simulink model "systemOffLine"  (Simulink 8.5)
settings: Solver=ode3  SolverMode=SingleTasking  StartTime=0.0  StopTime=0.1  RelTol=1e-3  AbsTol=1e-6
undefined symbols (not defined in the file or in its folder): DAB, den, elements, num
(part 5 of 5)

== system systemOffLine/Distance Relay Substation A2/Fault B-G Measurement/Zone R ==
  Z : Inport
  <V : Inport  Port=2
  " 5" : Fcn  Expr=sqrt(u)
  " 6" : RelationalOperator  Operator=<  OutDataTypeStr=boolean
  6 : Fcn  Expr=sqrt(u)
  Integrator : Integrator
  Product{,1..3} (4 alike) : Product  RndMeth=Zero
  "R, X" : Demux  Outputs=2
  Rdiff : Sum  Inputs=+-  SaturateOnIntegerOverflow=on  InputSameDT=on  OutDataTypeStr=Inherit: Same as first input
  Rr : Constant  Value=Rr/2
  Startup : Product  Inputs=3  RndMeth=Zero
  Step : Step  Time=0.017  SampleTime=0
  TRIP output contact : Relay  OnSwitchValue=0.9999  OffSwitchValue=-1
  Xdiff : Sum  Inputs=+-  SaturateOnIntegerOverflow=on  InputSameDT=on  OutDataTypeStr=Inherit: Same as first input
  Xr : Constant  Value=Xr/2
  Zm2 : Sum  SaturateOnIntegerOverflow=on  InputSameDT=on  OutDataTypeStr=Inherit: Same as first input
  Zr2 : Sum  SaturateOnIntegerOverflow=on  InputSameDT=on  OutDataTypeStr=Inherit: Same as first input
  delay : RelationalOperator  Operator=>  InputSameDT=on
  time delay : Constant  Value=Td+0.001
  TRIP : Outport  InitialOutput=0
  Zm : Outport  Port=2  InitialOutput=0
  Zr : Outport  Port=3  InitialOutput=0
  wires:
  Z/1 -> "R, X"/1
  Rr/1 -> Rdiff/1, Product1/2, Product1/1
  "R, X"/1 -> Rdiff/2
  "R, X"/2 -> Xdiff/1
  Xr/1 -> Xdiff/2, Product3/2, Product3/1
  Xdiff/1 -> Product2/2, Product2/1
  Product/1 -> Zm2/1
  Product2/1 -> Zm2/2
  Product1/1 -> Zr2/1
  Product3/1 -> Zr2/2
  Zm2/1 -> 6/1
  Zr2/1 -> " 5"/1
  6/1 -> " 6"/1, Zm/1
  " 5"/1 -> " 6"/2, Zr/1
  " 6"/1 -> Startup/1
  <V/1 -> Startup/3
  Step/1 -> Startup/2
  Rdiff/1 -> Product/1, Product/2
  Integrator/1 -> delay/1
  time delay/1 -> delay/2
  delay/1 -> TRIP output contact/1
  Startup/1 -> Integrator/1
  TRIP output contact/1 -> TRIP/1

== system systemOffLine/Distance Relay Substation A2/Fault C-A Measurement/Zone 1 ==
  Z : Inport
  <V : Inport  Port=2
  " 5" : Fcn  Expr=sqrt(u)
  " 6" : RelationalOperator  Operator=<  OutDataTypeStr=boolean
  6 : Fcn  Expr=sqrt(u)
  Integrator : Integrator
  Product{,1..3} (4 alike) : Product  RndMeth=Zero
  "R, X" : Demux  Outputs=2
  Rdiff : Sum  Inputs=+-  SaturateOnIntegerOverflow=on  InputSameDT=on  OutDataTypeStr=Inherit: Same as first input
  Rr : Constant  Value=Rr/2
  Startup : Product  Inputs=3  RndMeth=Zero
  Step : Step  Time=0.017  SampleTime=0
  TRIP output contact : Relay  OnSwitchValue=0.9999  OffSwitchValue=-1
  Xdiff : Sum  Inputs=+-  SaturateOnIntegerOverflow=on  InputSameDT=on  OutDataTypeStr=Inherit: Same as first input
  Xr : Constant  Value=Xr/2
  Zm2 : Sum  SaturateOnIntegerOverflow=on  InputSameDT=on  OutDataTypeStr=Inherit: Same as first input
  Zr2 : Sum  SaturateOnIntegerOverflow=on  InputSameDT=on  OutDataTypeStr=Inherit: Same as first input
  delay : RelationalOperator  Operator=>  InputSameDT=on
  time delay : Constant  Value=Td+0.001
  TRIP : Outport  InitialOutput=0
  Zm : Outport  Port=2  InitialOutput=0
  Zr : Outport  Port=3  InitialOutput=0
  wires:
  TRIP output contact/1 -> TRIP/1
  Startup/1 -> Integrator/1
  delay/1 -> TRIP output contact/1
  time delay/1 -> delay/2
  Integrator/1 -> delay/1
  Rdiff/1 -> Product/2, Product/1
  Step/1 -> Startup/2
  <V/1 -> Startup/3
  " 6"/1 -> Startup/1
  " 5"/1 -> Zr/1, " 6"/2
  6/1 -> Zm/1, " 6"/1
  Zr2/1 -> " 5"/1
  Zm2/1 -> 6/1
  Product3/1 -> Zr2/2
  Product1/1 -> Zr2/1
  Product2/1 -> Zm2/2
  Product/1 -> Zm2/1
  Xdiff/1 -> Product2/1, Product2/2
  Xr/1 -> Product3/1, Product3/2, Xdiff/2
  "R, X"/2 -> Xdiff/1
  "R, X"/1 -> Rdiff/2
  Rr/1 -> Product1/1, Product1/2, Rdiff/1
  Z/1 -> "R, X"/1

== system systemOffLine/Distance Relay Substation A2/Fault C-A Measurement/Zone 2 ==
  Z : Inport
  <V : Inport  Port=2
  " 5" : Fcn  Expr=sqrt(u)
  " 6" : RelationalOperator  Operator=<  OutDataTypeStr=boolean
  6 : Fcn  Expr=sqrt(u)
  Integrator : Integrator
  Product{,1..3} (4 alike) : Product  RndMeth=Zero
  "R, X" : Demux  Outputs=2
  Rdiff : Sum  Inputs=+-  SaturateOnIntegerOverflow=on  InputSameDT=on  OutDataTypeStr=Inherit: Same as first input
  Rr : Constant  Value=Rr/2
  Startup : Product  Inputs=3  RndMeth=Zero
  Step : Step  Time=0.017  SampleTime=0
  TRIP output contact : Relay  OnSwitchValue=0.9999  OffSwitchValue=-1
  Xdiff : Sum  Inputs=+-  SaturateOnIntegerOverflow=on  InputSameDT=on  OutDataTypeStr=Inherit: Same as first input
  Xr : Constant  Value=Xr/2
  Zm2 : Sum  SaturateOnIntegerOverflow=on  InputSameDT=on  OutDataTypeStr=Inherit: Same as first input
  Zr2 : Sum  SaturateOnIntegerOverflow=on  InputSameDT=on  OutDataTypeStr=Inherit: Same as first input
  delay : RelationalOperator  Operator=>  InputSameDT=on
  time delay : Constant  Value=Td+0.001
  TRIP : Outport  InitialOutput=0
  Zm : Outport  Port=2  InitialOutput=0
  Zr : Outport  Port=3  InitialOutput=0
  wires:
  Z/1 -> "R, X"/1
  Rr/1 -> Rdiff/1, Product1/2, Product1/1
  "R, X"/1 -> Rdiff/2
  "R, X"/2 -> Xdiff/1
  Xr/1 -> Xdiff/2, Product3/2, Product3/1
  Xdiff/1 -> Product2/2, Product2/1
  Product/1 -> Zm2/1
  Product2/1 -> Zm2/2
  Product1/1 -> Zr2/1
  Product3/1 -> Zr2/2
  Zm2/1 -> 6/1
  Zr2/1 -> " 5"/1
  6/1 -> " 6"/1, Zm/1
  " 5"/1 -> " 6"/2, Zr/1
  " 6"/1 -> Startup/1
  <V/1 -> Startup/3
  Step/1 -> Startup/2
  Rdiff/1 -> Product/1, Product/2
  Integrator/1 -> delay/1
  time delay/1 -> delay/2
  delay/1 -> TRIP output contact/1
  Startup/1 -> Integrator/1
  TRIP output contact/1 -> TRIP/1

== system systemOffLine/Distance Relay Substation A2/Fault C-A Measurement/Zone 3 ==
  Z : Inport
  <V : Inport  Port=2
  " 5" : Fcn  Expr=sqrt(u)
  " 6" : RelationalOperator  Operator=<  OutDataTypeStr=boolean
  6 : Fcn  Expr=sqrt(u)
  Integrator : Integrator
  Product{,1..3} (4 alike) : Product  RndMeth=Zero
  "R, X" : Demux  Outputs=2
  Rdiff : Sum  Inputs=+-  SaturateOnIntegerOverflow=on  InputSameDT=on  OutDataTypeStr=Inherit: Same as first input
  Rr : Constant  Value=-Rr/2
  Startup : Product  Inputs=3  RndMeth=Zero
  Step : Step  Time=0.017  SampleTime=0
  TRIP output contact : Relay  OnSwitchValue=0.9999  OffSwitchValue=-1
  Xdiff : Sum  Inputs=+-  SaturateOnIntegerOverflow=on  InputSameDT=on  OutDataTypeStr=Inherit: Same as first input
  Xr : Constant  Value=-Xr/2
  Zm2 : Sum  SaturateOnIntegerOverflow=on  InputSameDT=on  OutDataTypeStr=Inherit: Same as first input
  Zr2 : Sum  SaturateOnIntegerOverflow=on  InputSameDT=on  OutDataTypeStr=Inherit: Same as first input
  delay : RelationalOperator  Operator=>  InputSameDT=on
  time delay : Constant  Value=Td+0.001
  TRIP : Outport  InitialOutput=0
  Zm : Outport  Port=2  InitialOutput=0
  Zr : Outport  Port=3  InitialOutput=0
  wires:
  TRIP output contact/1 -> TRIP/1
  Startup/1 -> Integrator/1
  delay/1 -> TRIP output contact/1
  time delay/1 -> delay/2
  Integrator/1 -> delay/1
  Rdiff/1 -> Product/2, Product/1
  Step/1 -> Startup/2
  <V/1 -> Startup/3
  " 6"/1 -> Startup/1
  " 5"/1 -> Zr/1, " 6"/2
  6/1 -> Zm/1, " 6"/1
  Zr2/1 -> " 5"/1
  Zm2/1 -> 6/1
  Product3/1 -> Zr2/2
  Product1/1 -> Zr2/1
  Product2/1 -> Zm2/2
  Product/1 -> Zm2/1
  Xdiff/1 -> Product2/1, Product2/2
  Xr/1 -> Product3/1, Product3/2, Xdiff/2
  "R, X"/2 -> Xdiff/1
  "R, X"/1 -> Rdiff/2
  Rr/1 -> Product1/1, Product1/2, Rdiff/1
  Z/1 -> "R, X"/1

== system systemOffLine/Distance Relay Substation A2/Fault C-A Measurement/Zone 4 ==
  Z : Inport
  <V : Inport  Port=2
  " 5" : Fcn  Expr=sqrt(u)
  " 6" : RelationalOperator  Operator=<  OutDataTypeStr=boolean
  6 : Fcn  Expr=sqrt(u)
  Integrator : Integrator
  Product{,1..3} (4 alike) : Product  RndMeth=Zero
  "R, X" : Demux  Outputs=2
  Rdiff : Sum  Inputs=+-  SaturateOnIntegerOverflow=on  InputSameDT=on  OutDataTypeStr=Inherit: Same as first input
  Rr : Constant  Value=Rr/2
  Startup : Product  Inputs=3  RndMeth=Zero
  Step : Step  Time=0.017  SampleTime=0
  TRIP output contact : Relay  OnSwitchValue=0.9999  OffSwitchValue=-1
  Xdiff : Sum  Inputs=+-  SaturateOnIntegerOverflow=on  InputSameDT=on  OutDataTypeStr=Inherit: Same as first input
  Xr : Constant  Value=Xr/2
  Zm2 : Sum  SaturateOnIntegerOverflow=on  InputSameDT=on  OutDataTypeStr=Inherit: Same as first input
  Zr2 : Sum  SaturateOnIntegerOverflow=on  InputSameDT=on  OutDataTypeStr=Inherit: Same as first input
  delay : RelationalOperator  Operator=>  InputSameDT=on
  time delay : Constant  Value=Td+0.001
  TRIP : Outport  InitialOutput=0
  Zm : Outport  Port=2  InitialOutput=0
  Zr : Outport  Port=3  InitialOutput=0
  wires:
  Z/1 -> "R, X"/1
  Rr/1 -> Rdiff/1, Product1/2, Product1/1
  "R, X"/1 -> Rdiff/2
  "R, X"/2 -> Xdiff/1
  Xr/1 -> Xdiff/2, Product3/2, Product3/1
  Xdiff/1 -> Product2/2, Product2/1
  Product/1 -> Zm2/1
  Product2/1 -> Zm2/2
  Product1/1 -> Zr2/1
  Product3/1 -> Zr2/2
  Zm2/1 -> 6/1
  Zr2/1 -> " 5"/1
  6/1 -> " 6"/1, Zm/1
  " 5"/1 -> " 6"/2, Zr/1
  " 6"/1 -> Startup/1
  <V/1 -> Startup/3
  Step/1 -> Startup/2
  Rdiff/1 -> Product/1, Product/2
  Integrator/1 -> delay/1
  time delay/1 -> delay/2
  delay/1 -> TRIP output contact/1
  Startup/1 -> Integrator/1
  TRIP output contact/1 -> TRIP/1

== system systemOffLine/Distance Relay Substation A2/Fault C-A Measurement/Zone R ==
  Z : Inport
  <V : Inport  Port=2
  " 5" : Fcn  Expr=sqrt(u)
  " 6" : RelationalOperator  Operator=<  OutDataTypeStr=boolean
  6 : Fcn  Expr=sqrt(u)
  Integrator : Integrator
  Product{,1..3} (4 alike) : Product  RndMeth=Zero
  "R, X" : Demux  Outputs=2
  Rdiff : Sum  Inputs=+-  SaturateOnIntegerOverflow=on  InputSameDT=on  OutDataTypeStr=Inherit: Same as first input
  Rr : Constant  Value=Rr/2
  Startup : Product  Inputs=3  RndMeth=Zero
  Step : Step  Time=0.017  SampleTime=0
  TRIP output contact : Relay  OnSwitchValue=0.9999  OffSwitchValue=-1
  Xdiff : Sum  Inputs=+-  SaturateOnIntegerOverflow=on  InputSameDT=on  OutDataTypeStr=Inherit: Same as first input
  Xr : Constant  Value=Xr/2
  Zm2 : Sum  SaturateOnIntegerOverflow=on  InputSameDT=on  OutDataTypeStr=Inherit: Same as first input
  Zr2 : Sum  SaturateOnIntegerOverflow=on  InputSameDT=on  OutDataTypeStr=Inherit: Same as first input
  delay : RelationalOperator  Operator=>  InputSameDT=on
  time delay : Constant  Value=Td+0.001
  TRIP : Outport  InitialOutput=0
  Zm : Outport  Port=2  InitialOutput=0
  Zr : Outport  Port=3  InitialOutput=0
  wires:
  Z/1 -> "R, X"/1
  Rr/1 -> Rdiff/1, Product1/2, Product1/1
  "R, X"/1 -> Rdiff/2
  "R, X"/2 -> Xdiff/1
  Xr/1 -> Xdiff/2, Product3/2, Product3/1
  Xdiff/1 -> Product2/2, Product2/1
  Product/1 -> Zm2/1
  Product2/1 -> Zm2/2
  Product1/1 -> Zr2/1
  Product3/1 -> Zr2/2
  Zm2/1 -> 6/1
  Zr2/1 -> " 5"/1
  6/1 -> " 6"/1, Zm/1
  " 5"/1 -> " 6"/2, Zr/1
  " 6"/1 -> Startup/1
  <V/1 -> Startup/3
  Step/1 -> Startup/2
  Rdiff/1 -> Product/1, Product/2
  Integrator/1 -> delay/1
  time delay/1 -> delay/2
  delay/1 -> TRIP output contact/1
  Startup/1 -> Integrator/1
  TRIP output contact/1 -> TRIP/1

== system systemOffLine/Distance Relay Substation A2/Fault C-G Measurement/Zone 1 ==
  Z : Inport
  <V : Inport  Port=2
  " 5" : Fcn  Expr=sqrt(u)
  " 6" : RelationalOperator  Operator=<  OutDataTypeStr=boolean
  6 : Fcn  Expr=sqrt(u)
  Integrator : Integrator
  Product{,1..3} (4 alike) : Product  RndMeth=Zero
  "R, X" : Demux  Outputs=2
  Rdiff : Sum  Inputs=+-  SaturateOnIntegerOverflow=on  InputSameDT=on  OutDataTypeStr=Inherit: Same as first input
  Rr : Constant  Value=Rr/2
  Startup : Product  Inputs=3  RndMeth=Zero
  Step : Step  Time=0.017  SampleTime=0
  TRIP output contact : Relay  OnSwitchValue=0.9999  OffSwitchValue=-1
  Xdiff : Sum  Inputs=+-  SaturateOnIntegerOverflow=on  InputSameDT=on  OutDataTypeStr=Inherit: Same as first input
  Xr : Constant  Value=Xr/2
  Zm2 : Sum  SaturateOnIntegerOverflow=on  InputSameDT=on  OutDataTypeStr=Inherit: Same as first input
  Zr2 : Sum  SaturateOnIntegerOverflow=on  InputSameDT=on  OutDataTypeStr=Inherit: Same as first input
  delay : RelationalOperator  Operator=>  InputSameDT=on
  time delay : Constant  Value=Td+0.001
  TRIP : Outport  InitialOutput=0
  Zm : Outport  Port=2  InitialOutput=0
  Zr : Outport  Port=3  InitialOutput=0
  wires:
  TRIP output contact/1 -> TRIP/1
  Startup/1 -> Integrator/1
  delay/1 -> TRIP output contact/1
  time delay/1 -> delay/2
  Integrator/1 -> delay/1
  Rdiff/1 -> Product/2, Product/1
  Step/1 -> Startup/2
  <V/1 -> Startup/3
  " 6"/1 -> Startup/1
  " 5"/1 -> Zr/1, " 6"/2
  6/1 -> Zm/1, " 6"/1
  Zr2/1 -> " 5"/1
  Zm2/1 -> 6/1
  Product3/1 -> Zr2/2
  Product1/1 -> Zr2/1
  Product2/1 -> Zm2/2
  Product/1 -> Zm2/1
  Xdiff/1 -> Product2/1, Product2/2
  Xr/1 -> Product3/1, Product3/2, Xdiff/2
  "R, X"/2 -> Xdiff/1
  "R, X"/1 -> Rdiff/2
  Rr/1 -> Product1/1, Product1/2, Rdiff/1
  Z/1 -> "R, X"/1

== system systemOffLine/Distance Relay Substation A2/Fault C-G Measurement/Zone 2 ==
  Z : Inport
  <V : Inport  Port=2
  " 5" : Fcn  Expr=sqrt(u)
  " 6" : RelationalOperator  Operator=<  OutDataTypeStr=boolean
  6 : Fcn  Expr=sqrt(u)
  Integrator : Integrator
  Product{,1..3} (4 alike) : Product  RndMeth=Zero
  "R, X" : Demux  Outputs=2
  Rdiff : Sum  Inputs=+-  SaturateOnIntegerOverflow=on  InputSameDT=on  OutDataTypeStr=Inherit: Same as first input
  Rr : Constant  Value=Rr/2
  Startup : Product  Inputs=3  RndMeth=Zero
  Step : Step  Time=0.017  SampleTime=0
  TRIP output contact : Relay  OnSwitchValue=0.9999  OffSwitchValue=-1
  Xdiff : Sum  Inputs=+-  SaturateOnIntegerOverflow=on  InputSameDT=on  OutDataTypeStr=Inherit: Same as first input
  Xr : Constant  Value=Xr/2
  Zm2 : Sum  SaturateOnIntegerOverflow=on  InputSameDT=on  OutDataTypeStr=Inherit: Same as first input
  Zr2 : Sum  SaturateOnIntegerOverflow=on  InputSameDT=on  OutDataTypeStr=Inherit: Same as first input
  delay : RelationalOperator  Operator=>  InputSameDT=on
  time delay : Constant  Value=Td+0.001
  TRIP : Outport  InitialOutput=0
  Zm : Outport  Port=2  InitialOutput=0
  Zr : Outport  Port=3  InitialOutput=0
  wires:
  Z/1 -> "R, X"/1
  Rr/1 -> Rdiff/1, Product1/2, Product1/1
  "R, X"/1 -> Rdiff/2
  "R, X"/2 -> Xdiff/1
  Xr/1 -> Xdiff/2, Product3/2, Product3/1
  Xdiff/1 -> Product2/2, Product2/1
  Product/1 -> Zm2/1
  Product2/1 -> Zm2/2
  Product1/1 -> Zr2/1
  Product3/1 -> Zr2/2
  Zm2/1 -> 6/1
  Zr2/1 -> " 5"/1
  6/1 -> " 6"/1, Zm/1
  " 5"/1 -> " 6"/2, Zr/1
  " 6"/1 -> Startup/1
  <V/1 -> Startup/3
  Step/1 -> Startup/2
  Rdiff/1 -> Product/1, Product/2
  Integrator/1 -> delay/1
  time delay/1 -> delay/2
  delay/1 -> TRIP output contact/1
  Startup/1 -> Integrator/1
  TRIP output contact/1 -> TRIP/1

== system systemOffLine/Distance Relay Substation A2/Fault C-G Measurement/Zone 3 ==
  Z : Inport
  <V : Inport  Port=2
  " 5" : Fcn  Expr=sqrt(u)
  " 6" : RelationalOperator  Operator=<  OutDataTypeStr=boolean
  6 : Fcn  Expr=sqrt(u)
  Integrator : Integrator
  Product{,1..3} (4 alike) : Product  RndMeth=Zero
  "R, X" : Demux  Outputs=2
  Rdiff : Sum  Inputs=+-  SaturateOnIntegerOverflow=on  InputSameDT=on  OutDataTypeStr=Inherit: Same as first input
  Rr : Constant  Value=-Rr/2
  Startup : Product  Inputs=3  RndMeth=Zero
  Step : Step  Time=0.017  SampleTime=0
  TRIP output contact : Relay  OnSwitchValue=0.9999  OffSwitchValue=-1
  Xdiff : Sum  Inputs=+-  SaturateOnIntegerOverflow=on  InputSameDT=on  OutDataTypeStr=Inherit: Same as first input
  Xr : Constant  Value=-Xr/2
  Zm2 : Sum  SaturateOnIntegerOverflow=on  InputSameDT=on  OutDataTypeStr=Inherit: Same as first input
  Zr2 : Sum  SaturateOnIntegerOverflow=on  InputSameDT=on  OutDataTypeStr=Inherit: Same as first input
  delay : RelationalOperator  Operator=>  InputSameDT=on
  time delay : Constant  Value=Td+0.001
  TRIP : Outport  InitialOutput=0
  Zm : Outport  Port=2  InitialOutput=0
  Zr : Outport  Port=3  InitialOutput=0
  wires:
  TRIP output contact/1 -> TRIP/1
  Startup/1 -> Integrator/1
  delay/1 -> TRIP output contact/1
  time delay/1 -> delay/2
  Integrator/1 -> delay/1
  Rdiff/1 -> Product/2, Product/1
  Step/1 -> Startup/2
  <V/1 -> Startup/3
  " 6"/1 -> Startup/1
  " 5"/1 -> Zr/1, " 6"/2
  6/1 -> Zm/1, " 6"/1
  Zr2/1 -> " 5"/1
  Zm2/1 -> 6/1
  Product3/1 -> Zr2/2
  Product1/1 -> Zr2/1
  Product2/1 -> Zm2/2
  Product/1 -> Zm2/1
  Xdiff/1 -> Product2/1, Product2/2
  Xr/1 -> Product3/1, Product3/2, Xdiff/2
  "R, X"/2 -> Xdiff/1
  "R, X"/1 -> Rdiff/2
  Rr/1 -> Product1/1, Product1/2, Rdiff/1
  Z/1 -> "R, X"/1

== system systemOffLine/Distance Relay Substation A2/Fault C-G Measurement/Zone 4 ==
  Z : Inport
  <V : Inport  Port=2
  " 5" : Fcn  Expr=sqrt(u)
  " 6" : RelationalOperator  Operator=<  OutDataTypeStr=boolean
  6 : Fcn  Expr=sqrt(u)
  Integrator : Integrator
  Product{,1..3} (4 alike) : Product  RndMeth=Zero
  "R, X" : Demux  Outputs=2
  Rdiff : Sum  Inputs=+-  SaturateOnIntegerOverflow=on  InputSameDT=on  OutDataTypeStr=Inherit: Same as first input
  Rr : Constant  Value=Rr/2
  Startup : Product  Inputs=3  RndMeth=Zero
  Step : Step  Time=0.017  SampleTime=0
  TRIP output contact : Relay  OnSwitchValue=0.9999  OffSwitchValue=-1
  Xdiff : Sum  Inputs=+-  SaturateOnIntegerOverflow=on  InputSameDT=on  OutDataTypeStr=Inherit: Same as first input
  Xr : Constant  Value=Xr/2
  Zm2 : Sum  SaturateOnIntegerOverflow=on  InputSameDT=on  OutDataTypeStr=Inherit: Same as first input
  Zr2 : Sum  SaturateOnIntegerOverflow=on  InputSameDT=on  OutDataTypeStr=Inherit: Same as first input
  delay : RelationalOperator  Operator=>  InputSameDT=on
  time delay : Constant  Value=Td+0.001
  TRIP : Outport  InitialOutput=0
  Zm : Outport  Port=2  InitialOutput=0
  Zr : Outport  Port=3  InitialOutput=0
  wires:
  Z/1 -> "R, X"/1
  Rr/1 -> Rdiff/1, Product1/2, Product1/1
  "R, X"/1 -> Rdiff/2
  "R, X"/2 -> Xdiff/1
  Xr/1 -> Xdiff/2, Product3/2, Product3/1
  Xdiff/1 -> Product2/2, Product2/1
  Product/1 -> Zm2/1
  Product2/1 -> Zm2/2
  Product1/1 -> Zr2/1
  Product3/1 -> Zr2/2
  Zm2/1 -> 6/1
  Zr2/1 -> " 5"/1
  6/1 -> " 6"/1, Zm/1
  " 5"/1 -> " 6"/2, Zr/1
  " 6"/1 -> Startup/1
  <V/1 -> Startup/3
  Step/1 -> Startup/2
  Rdiff/1 -> Product/1, Product/2
  Integrator/1 -> delay/1
  time delay/1 -> delay/2
  delay/1 -> TRIP output contact/1
  Startup/1 -> Integrator/1
  TRIP output contact/1 -> TRIP/1

== system systemOffLine/Distance Relay Substation A2/Fault C-G Measurement/Zone R ==
  Z : Inport
  <V : Inport  Port=2
  " 5" : Fcn  Expr=sqrt(u)
  " 6" : RelationalOperator  Operator=<  OutDataTypeStr=boolean
  6 : Fcn  Expr=sqrt(u)
  Integrator : Integrator
  Product{,1..3} (4 alike) : Product  RndMeth=Zero
  "R, X" : Demux  Outputs=2
  Rdiff : Sum  Inputs=+-  SaturateOnIntegerOverflow=on  InputSameDT=on  OutDataTypeStr=Inherit: Same as first input
  Rr : Constant  Value=Rr/2
  Startup : Product  Inputs=3  RndMeth=Zero
  Step : Step  Time=0.017  SampleTime=0
  TRIP output contact : Relay  OnSwitchValue=0.9999  OffSwitchValue=-1
  Xdiff : Sum  Inputs=+-  SaturateOnIntegerOverflow=on  InputSameDT=on  OutDataTypeStr=Inherit: Same as first input
  Xr : Constant  Value=Xr/2
  Zm2 : Sum  SaturateOnIntegerOverflow=on  InputSameDT=on  OutDataTypeStr=Inherit: Same as first input
  Zr2 : Sum  SaturateOnIntegerOverflow=on  InputSameDT=on  OutDataTypeStr=Inherit: Same as first input
  delay : RelationalOperator  Operator=>  InputSameDT=on
  time delay : Constant  Value=Td+0.001
  TRIP : Outport  InitialOutput=0
  Zm : Outport  Port=2  InitialOutput=0
  Zr : Outport  Port=3  InitialOutput=0
  wires:
  Z/1 -> "R, X"/1
  Rr/1 -> Rdiff/1, Product1/2, Product1/1
  "R, X"/1 -> Rdiff/2
  "R, X"/2 -> Xdiff/1
  Xr/1 -> Xdiff/2, Product3/2, Product3/1
  Xdiff/1 -> Product2/2, Product2/1
  Product/1 -> Zm2/1
  Product2/1 -> Zm2/2
  Product1/1 -> Zr2/1
  Product3/1 -> Zr2/2
  Zm2/1 -> 6/1
  Zr2/1 -> " 5"/1
  6/1 -> " 6"/1, Zm/1
  " 5"/1 -> " 6"/2, Zr/1
  " 6"/1 -> Startup/1
  <V/1 -> Startup/3
  Step/1 -> Startup/2
  Rdiff/1 -> Product/1, Product/2
  Integrator/1 -> delay/1
  time delay/1 -> delay/2
  delay/1 -> TRIP output contact/1
  Startup/1 -> Integrator/1
  TRIP output contact/1 -> TRIP/1

== system systemOffLine/Distance Relay Substation A1/Analog filtering, signal  conditioning/CURRENTS/DAB - current A ==
  a : Inport
  Analog Filter : TransferFcn  Numerator=num  Denominator=den
  Gain : Gain  Gain=G  SaturateOnIntegerOverflow=on  OutDataTypeStr=Inherit: Same as input  ParamDataTypeStr=Inherit: Same as input
  d : Outport  InitialOutput=[zeros(winsize,1)]
  wires:
  a/1 -> Analog Filter/1
  Analog Filter/1 -> Gain/1
  Gain/1 -> d/1

== system systemOffLine/Distance Relay Substation A1/Analog filtering, signal  conditioning/CURRENTS/DAB - current B ==
  a : Inport
  Analog Filter : TransferFcn  Numerator=num  Denominator=den
  Gain : Gain  Gain=G  SaturateOnIntegerOverflow=on  OutDataTypeStr=Inherit: Same as input  ParamDataTypeStr=Inherit: Same as input
  d : Outport  InitialOutput=[zeros(winsize,1)]
  wires:
  Gain/1 -> d/1
  Analog Filter/1 -> Gain/1
  a/1 -> Analog Filter/1

== system systemOffLine/Distance Relay Substation A1/Analog filtering, signal  conditioning/CURRENTS/DAB - current C ==
  a : Inport
  Analog Filter : TransferFcn  Numerator=num  Denominator=den
  Gain : Gain  Gain=G  SaturateOnIntegerOverflow=on  OutDataTypeStr=Inherit: Same as input  ParamDataTypeStr=Inherit: Same as input
  d : Outport  InitialOutput=[zeros(winsize,1)]
  wires:
  a/1 -> Analog Filter/1
  Analog Filter/1 -> Gain/1
  Gain/1 -> d/1

== system systemOffLine/Distance Relay Substation A1/Analog filtering, signal  conditioning/CURRENTS/Phasor IA ==
  signal : Inport
  Fcn : Fcn  Expr=u^2
  Fcn1 : Fcn  Expr=u^2
  Fcn2 : Fcn  Expr=sqrt(u)
  Fcn3 : Fcn  Expr=180/pi*atan2(u[2],u[1])
  Gain1 : Gain  Gain=k*f1  SaturateOnIntegerOverflow=on  OutDataTypeStr=Inherit: Same as input  ParamDataTypeStr=Inherit: Same as input
  Integ2 : Integrator
  Mux : Mux  Inputs=2
  Product : Product  SaturateOnIntegerOverflow=on  InputSameDT=on  OutDataTypeStr=Inherit: Same as first input
  Product1 : Product  SaturateOnIntegerOverflow=on  InputSameDT=on  OutDataTypeStr=Inherit: Same as first input
  Sum : Sum  SaturateOnIntegerOverflow=on  InputSameDT=on  OutDataTypeStr=Inherit: Same as first input
  Sum1 : Sum  Inputs=+-  SaturateOnIntegerOverflow=on  InputSameDT=on  OutDataTypeStr=Inherit: Same as first input
  Sum2 : Sum  Inputs=+-  SaturateOnIntegerOverflow=on  InputSameDT=on  OutDataTypeStr=Inherit: Same as first input
  T1 : TransportDelay  DelayTime=1/f1  BufferSize=15360
  T2 : TransportDelay  DelayTime=1/f1  BufferSize=15360
  cos(nwt) : Sin  Frequency=2*pi*n*f1  Phase=pi/2  SampleTime=0
  integ1 : Integrator
  sin(nwt) : Sin  Frequency=2*pi*n*f1  SampleTime=0
  magnitude : Outport  InitialOutput=0
  angle : Outport  Port=2  InitialOutput=0
  wires:
  Sum/1 -> Fcn2/1
  Fcn/1 -> Sum/1
  Fcn1/1 -> Sum/2
  Mux/1 -> Fcn3/1
  Fcn3/1 -> angle/1
  sin(nwt)/1 -> Product/1
  cos(nwt)/1 -> Product1/2
  Product/1 -> integ1/1
  Product1/1 -> Integ2/1
  T1/1 -> Sum1/2
  T2/1 -> Sum2/2
  integ1/1 -> T1/1, Sum1/1
  Integ2/1 -> T2/1, Sum2/1
  Sum2/1 -> Fcn1/1, Mux/2
  Sum1/1 -> Fcn/1, Mux/1
  signal/1 -> Gain1/1
  Gain1/1 -> Product/2, Product1/1
  Fcn2/1 -> magnitude/1

== system systemOffLine/Distance Relay Substation A1/Analog filtering, signal  conditioning/CURRENTS/Phasor IB ==
  signal : Inport
  Fcn : Fcn  Expr=u^2
  Fcn1 : Fcn  Expr=u^2
  Fcn2 : Fcn  Expr=sqrt(u)
  Fcn3 : Fcn  Expr=180/pi*atan2(u[2],u[1])
  Gain1 : Gain  Gain=k*f1  SaturateOnIntegerOverflow=on  OutDataTypeStr=Inherit: Same as input  ParamDataTypeStr=Inherit: Same as input
  Integ2 : Integrator
  Mux : Mux  Inputs=2
  Product : Product  SaturateOnIntegerOverflow=on  InputSameDT=on  OutDataTypeStr=Inherit: Same as first input
  Product1 : Product  SaturateOnIntegerOverflow=on  InputSameDT=on  OutDataTypeStr=Inherit: Same as first input
  Sum : Sum  SaturateOnIntegerOverflow=on  InputSameDT=on  OutDataTypeStr=Inherit: Same as first input
  Sum1 : Sum  Inputs=+-  SaturateOnIntegerOverflow=on  InputSameDT=on  OutDataTypeStr=Inherit: Same as first input
  Sum2 : Sum  Inputs=+-  SaturateOnIntegerOverflow=on  InputSameDT=on  OutDataTypeStr=Inherit: Same as first input
  T1 : TransportDelay  DelayTime=1/f1  BufferSize=15360
  T2 : TransportDelay  DelayTime=1/f1  BufferSize=15360
  cos(nwt) : Sin  Frequency=2*pi*n*f1  Phase=pi/2  SampleTime=0
  integ1 : Integrator
  sin(nwt) : Sin  Frequency=2*pi*n*f1  SampleTime=0
  magnitude : Outport  InitialOutput=0
  angle : Outport  Port=2  InitialOutput=0
  wires:
  Fcn2/1 -> magnitude/1
  Gain1/1 -> Product1/1, Product/2
  signal/1 -> Gain1/1
  Sum1/1 -> Mux/1, Fcn/1
  Sum2/1 -> Mux/2, Fcn1/1
  Integ2/1 -> Sum2/1, T2/1
  integ1/1 -> Sum1/1, T1/1
  T2/1 -> Sum2/2
  T1/1 -> Sum1/2
  Product1/1 -> Integ2/1
  Product/1 -> integ1/1
  cos(nwt)/1 -> Product1/2
  sin(nwt)/1 -> Product/1
  Fcn3/1 -> angle/1
  Mux/1 -> Fcn3/1
  Fcn1/1 -> Sum/2
  Fcn/1 -> Sum/1
  Sum/1 -> Fcn2/1

== system systemOffLine/Distance Relay Substation A1/Analog filtering, signal  conditioning/CURRENTS/Phasor IC ==
  signal : Inport
  Fcn : Fcn  Expr=u^2
  Fcn1 : Fcn  Expr=u^2
  Fcn2 : Fcn  Expr=sqrt(u)
  Fcn3 : Fcn  Expr=180/pi*atan2(u[2],u[1])
  Gain1 : Gain  Gain=k*f1  SaturateOnIntegerOverflow=on  OutDataTypeStr=Inherit: Same as input  ParamDataTypeStr=Inherit: Same as input
  Integ2 : Integrator
  Mux : Mux  Inputs=2
  Product : Product  SaturateOnIntegerOverflow=on  InputSameDT=on  OutDataTypeStr=Inherit: Same as first input
  Product1 : Product  SaturateOnIntegerOverflow=on  InputSameDT=on  OutDataTypeStr=Inherit: Same as first input
  Sum : Sum  SaturateOnIntegerOverflow=on  InputSameDT=on  OutDataTypeStr=Inherit: Same as first input
  Sum1 : Sum  Inputs=+-  SaturateOnIntegerOverflow=on  InputSameDT=on  OutDataTypeStr=Inherit: Same as first input
  Sum2 : Sum  Inputs=+-  SaturateOnIntegerOverflow=on  InputSameDT=on  OutDataTypeStr=Inherit: Same as first input
  T1 : TransportDelay  DelayTime=1/f1  BufferSize=15360
  T2 : TransportDelay  DelayTime=1/f1  BufferSize=15360
  cos(nwt) : Sin  Frequency=2*pi*n*f1  Phase=pi/2  SampleTime=0
  integ1 : Integrator
  sin(nwt) : Sin  Frequency=2*pi*n*f1  SampleTime=0
  magnitude : Outport  InitialOutput=0
  angle : Outport  Port=2  InitialOutput=0
  wires:
  Sum/1 -> Fcn2/1
  Fcn/1 -> Sum/1
  Fcn1/1 -> Sum/2
  Mux/1 -> Fcn3/1
  Fcn3/1 -> angle/1
  sin(nwt)/1 -> Product/1
  cos(nwt)/1 -> Product1/2
  Product/1 -> integ1/1
  Product1/1 -> Integ2/1
  T1/1 -> Sum1/2
  T2/1 -> Sum2/2
  integ1/1 -> T1/1, Sum1/1
  Integ2/1 -> T2/1, Sum2/1
  Sum2/1 -> Fcn1/1, Mux/2
  Sum1/1 -> Fcn/1, Mux/1
  signal/1 -> Gain1/1
  Gain1/1 -> Product/2, Product1/1
  Fcn2/1 -> magnitude/1

== system systemOffLine/Distance Relay Substation A1/Analog filtering, signal  conditioning/VOLTAGES/DAB - voltage A ==
  a : Inport
  Analog Filter : TransferFcn  Numerator=num  Denominator=den
  Gain : Gain  Gain=G  SaturateOnIntegerOverflow=on  OutDataTypeStr=Inherit: Same as input  ParamDataTypeStr=Inherit: Same as input
  d : Outport  InitialOutput=[zeros(winsize,1)]
  wires:
  Gain/1 -> d/1
  Analog Filter/1 -> Gain/1
  a/1 -> Analog Filter/1

== system systemOffLine/Distance Relay Substation A1/Analog filtering, signal  conditioning/VOLTAGES/DAB - voltage B ==
  a : Inport
  Analog Filter : TransferFcn  Numerator=num  Denominator=den
  Gain : Gain  Gain=G  SaturateOnIntegerOverflow=on  OutDataTypeStr=Inherit: Same as input  ParamDataTypeStr=Inherit: Same as input
  d : Outport  InitialOutput=[zeros(winsize,1)]
  wires:
  a/1 -> Analog Filter/1
  Analog Filter/1 -> Gain/1
  Gain/1 -> d/1

== system systemOffLine/Distance Relay Substation A1/Analog filtering, signal  conditioning/VOLTAGES/DAB - voltage C ==
  a : Inport
  Analog Filter : TransferFcn  Numerator=num  Denominator=den
  Gain : Gain  Gain=G  SaturateOnIntegerOverflow=on  OutDataTypeStr=Inherit: Same as input  ParamDataTypeStr=Inherit: Same as input
  d : Outport  InitialOutput=[zeros(winsize,1)]
  wires:
  Gain/1 -> d/1
  Analog Filter/1 -> Gain/1
  a/1 -> Analog Filter/1

== system systemOffLine/Distance Relay Substation A1/Analog filtering, signal  conditioning/VOLTAGES/Phasor VA ==
  signal : Inport
  Fcn : Fcn  Expr=u^2
  Fcn1 : Fcn  Expr=u^2
  Fcn2 : Fcn  Expr=sqrt(u)
  Fcn3 : Fcn  Expr=180/pi*atan2(u[2],u[1])
  Gain1 : Gain  Gain=k*f1  SaturateOnIntegerOverflow=on  OutDataTypeStr=Inherit: Same as input  ParamDataTypeStr=Inherit: Same as input
  Integ2 : Integrator
  Mux : Mux  Inputs=2
  Product : Product  SaturateOnIntegerOverflow=on  InputSameDT=on  OutDataTypeStr=Inherit: Same as first input
  Product1 : Product  SaturateOnIntegerOverflow=on  InputSameDT=on  OutDataTypeStr=Inherit: Same as first input
  Sum : Sum  SaturateOnIntegerOverflow=on  InputSameDT=on  OutDataTypeStr=Inherit: Same as first input
  Sum1 : Sum  Inputs=+-  SaturateOnIntegerOverflow=on  InputSameDT=on  OutDataTypeStr=Inherit: Same as first input
  Sum2 : Sum  Inputs=+-  SaturateOnIntegerOverflow=on  InputSameDT=on  OutDataTypeStr=Inherit: Same as first input
  T1 : TransportDelay  DelayTime=1/f1  BufferSize=15360
  T2 : TransportDelay  DelayTime=1/f1  BufferSize=15360
  cos(nwt) : Sin  Frequency=2*pi*n*f1  Phase=pi/2  SampleTime=0
  integ1 : Integrator
  sin(nwt) : Sin  Frequency=2*pi*n*f1  SampleTime=0
  magnitude : Outport  InitialOutput=0
  angle : Outport  Port=2  InitialOutput=0
  wires:
  Sum/1 -> Fcn2/1
  Fcn/1 -> Sum/1
  Fcn1/1 -> Sum/2
  Mux/1 -> Fcn3/1
  Fcn3/1 -> angle/1
  sin(nwt)/1 -> Product/1
  cos(nwt)/1 -> Product1/2
  Product/1 -> integ1/1
  Product1/1 -> Integ2/1
  T1/1 -> Sum1/2
  T2/1 -> Sum2/2
  integ1/1 -> T1/1, Sum1/1
  Integ2/1 -> T2/1, Sum2/1
  Sum2/1 -> Fcn1/1, Mux/2
  Sum1/1 -> Fcn/1, Mux/1
  signal/1 -> Gain1/1
  Gain1/1 -> Product/2, Product1/1
  Fcn2/1 -> magnitude/1

== system systemOffLine/Distance Relay Substation A1/Analog filtering, signal  conditioning/VOLTAGES/Phasor VB ==
  signal : Inport
  Fcn : Fcn  Expr=u^2
  Fcn1 : Fcn  Expr=u^2
  Fcn2 : Fcn  Expr=sqrt(u)
  Fcn3 : Fcn  Expr=180/pi*atan2(u[2],u[1])
  Gain1 : Gain  Gain=k*f1  SaturateOnIntegerOverflow=on  OutDataTypeStr=Inherit: Same as input  ParamDataTypeStr=Inherit: Same as input
  Integ2 : Integrator
  Mux : Mux  Inputs=2
  Product : Product  SaturateOnIntegerOverflow=on  InputSameDT=on  OutDataTypeStr=Inherit: Same as first input
  Product1 : Product  SaturateOnIntegerOverflow=on  InputSameDT=on  OutDataTypeStr=Inherit: Same as first input
  Sum : Sum  SaturateOnIntegerOverflow=on  InputSameDT=on  OutDataTypeStr=Inherit: Same as first input
  Sum1 : Sum  Inputs=+-  SaturateOnIntegerOverflow=on  InputSameDT=on  OutDataTypeStr=Inherit: Same as first input
  Sum2 : Sum  Inputs=+-  SaturateOnIntegerOverflow=on  InputSameDT=on  OutDataTypeStr=Inherit: Same as first input
  T1 : TransportDelay  DelayTime=1/f1  BufferSize=15360
  T2 : TransportDelay  DelayTime=1/f1  BufferSize=15360
  cos(nwt) : Sin  Frequency=2*pi*n*f1  Phase=pi/2  SampleTime=0
  integ1 : Integrator
  sin(nwt) : Sin  Frequency=2*pi*n*f1  SampleTime=0
  magnitude : Outport  InitialOutput=0
  angle : Outport  Port=2  InitialOutput=0
  wires:
  Fcn2/1 -> magnitude/1
  Gain1/1 -> Product1/1, Product/2
  signal/1 -> Gain1/1
  Sum1/1 -> Mux/1, Fcn/1
  Sum2/1 -> Mux/2, Fcn1/1
  Integ2/1 -> Sum2/1, T2/1
  integ1/1 -> Sum1/1, T1/1
  T2/1 -> Sum2/2
  T1/1 -> Sum1/2
  Product1/1 -> Integ2/1
  Product/1 -> integ1/1
  cos(nwt)/1 -> Product1/2
  sin(nwt)/1 -> Product/1
  Fcn3/1 -> angle/1
  Mux/1 -> Fcn3/1
  Fcn1/1 -> Sum/2
  Fcn/1 -> Sum/1
  Sum/1 -> Fcn2/1

== system systemOffLine/Distance Relay Substation A1/Analog filtering, signal  conditioning/VOLTAGES/Phasor VC ==
  signal : Inport
  Fcn : Fcn  Expr=u^2
  Fcn1 : Fcn  Expr=u^2
  Fcn2 : Fcn  Expr=sqrt(u)
  Fcn3 : Fcn  Expr=180/pi*atan2(u[2],u[1])
  Gain1 : Gain  Gain=k*f1  SaturateOnIntegerOverflow=on  OutDataTypeStr=Inherit: Same as input  ParamDataTypeStr=Inherit: Same as input
  Integ2 : Integrator
  Mux : Mux  Inputs=2
  Product : Product  SaturateOnIntegerOverflow=on  InputSameDT=on  OutDataTypeStr=Inherit: Same as first input
  Product1 : Product  SaturateOnIntegerOverflow=on  InputSameDT=on  OutDataTypeStr=Inherit: Same as first input
  Sum : Sum  SaturateOnIntegerOverflow=on  InputSameDT=on  OutDataTypeStr=Inherit: Same as first input
  Sum1 : Sum  Inputs=+-  SaturateOnIntegerOverflow=on  InputSameDT=on  OutDataTypeStr=Inherit: Same as first input
  Sum2 : Sum  Inputs=+-  SaturateOnIntegerOverflow=on  InputSameDT=on  OutDataTypeStr=Inherit: Same as first input
  T1 : TransportDelay  DelayTime=1/f1  BufferSize=15360
  T2 : TransportDelay  DelayTime=1/f1  BufferSize=15360
  cos(nwt) : Sin  Frequency=2*pi*n*f1  Phase=pi/2  SampleTime=0
  integ1 : Integrator
  sin(nwt) : Sin  Frequency=2*pi*n*f1  SampleTime=0
  magnitude : Outport  InitialOutput=0
  angle : Outport  Port=2  InitialOutput=0
  wires:
  Sum/1 -> Fcn2/1
  Fcn/1 -> Sum/1
  Fcn1/1 -> Sum/2
  Mux/1 -> Fcn3/1
  Fcn3/1 -> angle/1
  sin(nwt)/1 -> Product/1
  cos(nwt)/1 -> Product1/2
  Product/1 -> integ1/1
  Product1/1 -> Integ2/1
  T1/1 -> Sum1/2
  T2/1 -> Sum2/2
  integ1/1 -> T1/1, Sum1/1
  Integ2/1 -> T2/1, Sum2/1
  Sum2/1 -> Fcn1/1, Mux/2
  Sum1/1 -> Fcn/1, Mux/1
  signal/1 -> Gain1/1
  Gain1/1 -> Product/2, Product1/1
  Fcn2/1 -> magnitude/1

== system systemOffLine/Distance Relay Substation A2/Analog filtering, signal  conditioning/CURRENTS/DAB - current A ==
  a : Inport
  Analog Filter : TransferFcn  Numerator=num  Denominator=den
  Gain : Gain  Gain=G  SaturateOnIntegerOverflow=on  OutDataTypeStr=Inherit: Same as input  ParamDataTypeStr=Inherit: Same as input
  d : Outport  InitialOutput=[zeros(winsize,1)]
  wires:
  a/1 -> Analog Filter/1
  Analog Filter/1 -> Gain/1
  Gain/1 -> d/1

== system systemOffLine/Distance Relay Substation A2/Analog filtering, signal  conditioning/CURRENTS/DAB - current B ==
  a : Inport
  Analog Filter : TransferFcn  Numerator=num  Denominator=den
  Gain : Gain  Gain=G  SaturateOnIntegerOverflow=on  OutDataTypeStr=Inherit: Same as input  ParamDataTypeStr=Inherit: Same as input
  d : Outport  InitialOutput=[zeros(winsize,1)]
  wires:
  Gain/1 -> d/1
  Analog Filter/1 -> Gain/1
  a/1 -> Analog Filter/1

== system systemOffLine/Distance Relay Substation A2/Analog filtering, signal  conditioning/CURRENTS/DAB - current C ==
  a : Inport
  Analog Filter : TransferFcn  Numerator=num  Denominator=den
  Gain : Gain  Gain=G  SaturateOnIntegerOverflow=on  OutDataTypeStr=Inherit: Same as input  ParamDataTypeStr=Inherit: Same as input
  d : Outport  InitialOutput=[zeros(winsize,1)]
  wires:
  a/1 -> Analog Filter/1
  Analog Filter/1 -> Gain/1
  Gain/1 -> d/1

== system systemOffLine/Distance Relay Substation A2/Analog filtering, signal  conditioning/CURRENTS/Phasor IA ==
  signal : Inport
  Fcn : Fcn  Expr=u^2
  Fcn1 : Fcn  Expr=u^2
  Fcn2 : Fcn  Expr=sqrt(u)
  Fcn3 : Fcn  Expr=180/pi*atan2(u[2],u[1])
  Gain1 : Gain  Gain=k*f1  SaturateOnIntegerOverflow=on  OutDataTypeStr=Inherit: Same as input  ParamDataTypeStr=Inherit: Same as input
  Integ2 : Integrator
  Mux : Mux  Inputs=2
  Product : Product  SaturateOnIntegerOverflow=on  InputSameDT=on  OutDataTypeStr=Inherit: Same as first input
  Product1 : Product  SaturateOnIntegerOverflow=on  InputSameDT=on  OutDataTypeStr=Inherit: Same as first input
  Sum : Sum  SaturateOnIntegerOverflow=on  InputSameDT=on  OutDataTypeStr=Inherit: Same as first input
  Sum1 : Sum  Inputs=+-  SaturateOnIntegerOverflow=on  InputSameDT=on  OutDataTypeStr=Inherit: Same as first input
  Sum2 : Sum  Inputs=+-  SaturateOnIntegerOverflow=on  InputSameDT=on  OutDataTypeStr=Inherit: Same as first input
  T1 : TransportDelay  DelayTime=1/f1  BufferSize=15360
  T2 : TransportDelay  DelayTime=1/f1  BufferSize=15360
  cos(nwt) : Sin  Frequency=2*pi*n*f1  Phase=pi/2  SampleTime=0
  integ1 : Integrator
  sin(nwt) : Sin  Frequency=2*pi*n*f1  SampleTime=0
  magnitude : Outport  InitialOutput=0
  angle : Outport  Port=2  InitialOutput=0
  wires:
  Sum/1 -> Fcn2/1
  Fcn/1 -> Sum/1
  Fcn1/1 -> Sum/2
  Mux/1 -> Fcn3/1
  Fcn3/1 -> angle/1
  sin(nwt)/1 -> Product/1
  cos(nwt)/1 -> Product1/2
  Product/1 -> integ1/1
  Product1/1 -> Integ2/1
  T1/1 -> Sum1/2
  T2/1 -> Sum2/2
  integ1/1 -> T1/1, Sum1/1
  Integ2/1 -> T2/1, Sum2/1
  Sum2/1 -> Fcn1/1, Mux/2
  Sum1/1 -> Fcn/1, Mux/1
  signal/1 -> Gain1/1
  Gain1/1 -> Product/2, Product1/1
  Fcn2/1 -> magnitude/1

== system systemOffLine/Distance Relay Substation A2/Analog filtering, signal  conditioning/CURRENTS/Phasor IB ==
  signal : Inport
  Fcn : Fcn  Expr=u^2
  Fcn1 : Fcn  Expr=u^2
  Fcn2 : Fcn  Expr=sqrt(u)
  Fcn3 : Fcn  Expr=180/pi*atan2(u[2],u[1])
  Gain1 : Gain  Gain=k*f1  SaturateOnIntegerOverflow=on  OutDataTypeStr=Inherit: Same as input  ParamDataTypeStr=Inherit: Same as input
  Integ2 : Integrator
  Mux : Mux  Inputs=2
  Product : Product  SaturateOnIntegerOverflow=on  InputSameDT=on  OutDataTypeStr=Inherit: Same as first input
  Product1 : Product  SaturateOnIntegerOverflow=on  InputSameDT=on  OutDataTypeStr=Inherit: Same as first input
  Sum : Sum  SaturateOnIntegerOverflow=on  InputSameDT=on  OutDataTypeStr=Inherit: Same as first input
  Sum1 : Sum  Inputs=+-  SaturateOnIntegerOverflow=on  InputSameDT=on  OutDataTypeStr=Inherit: Same as first input
  Sum2 : Sum  Inputs=+-  SaturateOnIntegerOverflow=on  InputSameDT=on  OutDataTypeStr=Inherit: Same as first input
  T1 : TransportDelay  DelayTime=1/f1  BufferSize=15360
  T2 : TransportDelay  DelayTime=1/f1  BufferSize=15360
  cos(nwt) : Sin  Frequency=2*pi*n*f1  Phase=pi/2  SampleTime=0
  integ1 : Integrator
  sin(nwt) : Sin  Frequency=2*pi*n*f1  SampleTime=0
  magnitude : Outport  InitialOutput=0
  angle : Outport  Port=2  InitialOutput=0
  wires:
  Fcn2/1 -> magnitude/1
  Gain1/1 -> Product1/1, Product/2
  signal/1 -> Gain1/1
  Sum1/1 -> Mux/1, Fcn/1
  Sum2/1 -> Mux/2, Fcn1/1
  Integ2/1 -> Sum2/1, T2/1
  integ1/1 -> Sum1/1, T1/1
  T2/1 -> Sum2/2
  T1/1 -> Sum1/2
  Product1/1 -> Integ2/1
  Product/1 -> integ1/1
  cos(nwt)/1 -> Product1/2
  sin(nwt)/1 -> Product/1
  Fcn3/1 -> angle/1
  Mux/1 -> Fcn3/1
  Fcn1/1 -> Sum/2
  Fcn/1 -> Sum/1
  Sum/1 -> Fcn2/1

== system systemOffLine/Distance Relay Substation A2/Analog filtering, signal  conditioning/CURRENTS/Phasor IC ==
  signal : Inport
  Fcn : Fcn  Expr=u^2
  Fcn1 : Fcn  Expr=u^2
  Fcn2 : Fcn  Expr=sqrt(u)
  Fcn3 : Fcn  Expr=180/pi*atan2(u[2],u[1])
  Gain1 : Gain  Gain=k*f1  SaturateOnIntegerOverflow=on  OutDataTypeStr=Inherit: Same as input  ParamDataTypeStr=Inherit: Same as input
  Integ2 : Integrator
  Mux : Mux  Inputs=2
  Product : Product  SaturateOnIntegerOverflow=on  InputSameDT=on  OutDataTypeStr=Inherit: Same as first input
  Product1 : Product  SaturateOnIntegerOverflow=on  InputSameDT=on  OutDataTypeStr=Inherit: Same as first input
  Sum : Sum  SaturateOnIntegerOverflow=on  InputSameDT=on  OutDataTypeStr=Inherit: Same as first input
  Sum1 : Sum  Inputs=+-  SaturateOnIntegerOverflow=on  InputSameDT=on  OutDataTypeStr=Inherit: Same as first input
  Sum2 : Sum  Inputs=+-  SaturateOnIntegerOverflow=on  InputSameDT=on  OutDataTypeStr=Inherit: Same as first input
  T1 : TransportDelay  DelayTime=1/f1  BufferSize=15360
  T2 : TransportDelay  DelayTime=1/f1  BufferSize=15360
  cos(nwt) : Sin  Frequency=2*pi*n*f1  Phase=pi/2  SampleTime=0
  integ1 : Integrator
  sin(nwt) : Sin  Frequency=2*pi*n*f1  SampleTime=0
  magnitude : Outport  InitialOutput=0
  angle : Outport  Port=2  InitialOutput=0
  wires:
  Sum/1 -> Fcn2/1
  Fcn/1 -> Sum/1
  Fcn1/1 -> Sum/2
  Mux/1 -> Fcn3/1
  Fcn3/1 -> angle/1
  sin(nwt)/1 -> Product/1
  cos(nwt)/1 -> Product1/2
  Product/1 -> integ1/1
  Product1/1 -> Integ2/1
  T1/1 -> Sum1/2
  T2/1 -> Sum2/2
  integ1/1 -> T1/1, Sum1/1
  Integ2/1 -> T2/1, Sum2/1
  Sum2/1 -> Fcn1/1, Mux/2
  Sum1/1 -> Fcn/1, Mux/1
  signal/1 -> Gain1/1
  Gain1/1 -> Product/2, Product1/1
  Fcn2/1 -> magnitude/1

== system systemOffLine/Distance Relay Substation A2/Analog filtering, signal  conditioning/VOLTAGES/DAB - voltage A ==
  a : Inport
  Analog Filter : TransferFcn  Numerator=num  Denominator=den
  Gain : Gain  Gain=G  SaturateOnIntegerOverflow=on  OutDataTypeStr=Inherit: Same as input  ParamDataTypeStr=Inherit: Same as input
  d : Outport  InitialOutput=[zeros(winsize,1)]
  wires:
  Gain/1 -> d/1
  Analog Filter/1 -> Gain/1
  a/1 -> Analog Filter/1

== system systemOffLine/Distance Relay Substation A2/Analog filtering, signal  conditioning/VOLTAGES/DAB - voltage B ==
  a : Inport
  Analog Filter : TransferFcn  Numerator=num  Denominator=den
  Gain : Gain  Gain=G  SaturateOnIntegerOverflow=on  OutDataTypeStr=Inherit: Same as input  ParamDataTypeStr=Inherit: Same as input
  d : Outport  InitialOutput=[zeros(winsize,1)]
  wires:
  a/1 -> Analog Filter/1
  Analog Filter/1 -> Gain/1
  Gain/1 -> d/1

== system systemOffLine/Distance Relay Substation A2/Analog filtering, signal  conditioning/VOLTAGES/DAB - voltage C ==
  a : Inport
  Analog Filter : TransferFcn  Numerator=num  Denominator=den
  Gain : Gain  Gain=G  SaturateOnIntegerOverflow=on  OutDataTypeStr=Inherit: Same as input  ParamDataTypeStr=Inherit: Same as input
  d : Outport  InitialOutput=[zeros(winsize,1)]
  wires:
  Gain/1 -> d/1
  Analog Filter/1 -> Gain/1
  a/1 -> Analog Filter/1

== system systemOffLine/Distance Relay Substation A2/Analog filtering, signal  conditioning/VOLTAGES/Phasor VA ==
  signal : Inport
  Fcn : Fcn  Expr=u^2
  Fcn1 : Fcn  Expr=u^2
  Fcn2 : Fcn  Expr=sqrt(u)
  Fcn3 : Fcn  Expr=180/pi*atan2(u[2],u[1])
  Gain1 : Gain  Gain=k*f1  SaturateOnIntegerOverflow=on  OutDataTypeStr=Inherit: Same as input  ParamDataTypeStr=Inherit: Same as input
  Integ2 : Integrator
  Mux : Mux  Inputs=2
  Product : Product  SaturateOnIntegerOverflow=on  InputSameDT=on  OutDataTypeStr=Inherit: Same as first input
  Product1 : Product  SaturateOnIntegerOverflow=on  InputSameDT=on  OutDataTypeStr=Inherit: Same as first input
  Sum : Sum  SaturateOnIntegerOverflow=on  InputSameDT=on  OutDataTypeStr=Inherit: Same as first input
  Sum1 : Sum  Inputs=+-  SaturateOnIntegerOverflow=on  InputSameDT=on  OutDataTypeStr=Inherit: Same as first input
  Sum2 : Sum  Inputs=+-  SaturateOnIntegerOverflow=on  InputSameDT=on  OutDataTypeStr=Inherit: Same as first input
  T1 : TransportDelay  DelayTime=1/f1  BufferSize=15360
  T2 : TransportDelay  DelayTime=1/f1  BufferSize=15360
  cos(nwt) : Sin  Frequency=2*pi*n*f1  Phase=pi/2  SampleTime=0
  integ1 : Integrator
  sin(nwt) : Sin  Frequency=2*pi*n*f1  SampleTime=0
  magnitude : Outport  InitialOutput=0
  angle : Outport  Port=2  InitialOutput=0
  wires:
  Sum/1 -> Fcn2/1
  Fcn/1 -> Sum/1
  Fcn1/1 -> Sum/2
  Mux/1 -> Fcn3/1
  Fcn3/1 -> angle/1
  sin(nwt)/1 -> Product/1
  cos(nwt)/1 -> Product1/2
  Product/1 -> integ1/1
  Product1/1 -> Integ2/1
  T1/1 -> Sum1/2
  T2/1 -> Sum2/2
  integ1/1 -> T1/1, Sum1/1
  Integ2/1 -> T2/1, Sum2/1
  Sum2/1 -> Fcn1/1, Mux/2
  Sum1/1 -> Fcn/1, Mux/1
  signal/1 -> Gain1/1
  Gain1/1 -> Product/2, Product1/1
  Fcn2/1 -> magnitude/1

== system systemOffLine/Distance Relay Substation A2/Analog filtering, signal  conditioning/VOLTAGES/Phasor VB ==
  signal : Inport
  Fcn : Fcn  Expr=u^2
  Fcn1 : Fcn  Expr=u^2
  Fcn2 : Fcn  Expr=sqrt(u)
  Fcn3 : Fcn  Expr=180/pi*atan2(u[2],u[1])
  Gain1 : Gain  Gain=k*f1  SaturateOnIntegerOverflow=on  OutDataTypeStr=Inherit: Same as input  ParamDataTypeStr=Inherit: Same as input
  Integ2 : Integrator
  Mux : Mux  Inputs=2
  Product : Product  SaturateOnIntegerOverflow=on  InputSameDT=on  OutDataTypeStr=Inherit: Same as first input
  Product1 : Product  SaturateOnIntegerOverflow=on  InputSameDT=on  OutDataTypeStr=Inherit: Same as first input
  Sum : Sum  SaturateOnIntegerOverflow=on  InputSameDT=on  OutDataTypeStr=Inherit: Same as first input
  Sum1 : Sum  Inputs=+-  SaturateOnIntegerOverflow=on  InputSameDT=on  OutDataTypeStr=Inherit: Same as first input
  Sum2 : Sum  Inputs=+-  SaturateOnIntegerOverflow=on  InputSameDT=on  OutDataTypeStr=Inherit: Same as first input
  T1 : TransportDelay  DelayTime=1/f1  BufferSize=15360
  T2 : TransportDelay  DelayTime=1/f1  BufferSize=15360
  cos(nwt) : Sin  Frequency=2*pi*n*f1  Phase=pi/2  SampleTime=0
  integ1 : Integrator
  sin(nwt) : Sin  Frequency=2*pi*n*f1  SampleTime=0
  magnitude : Outport  InitialOutput=0
  angle : Outport  Port=2  InitialOutput=0
  wires:
  Fcn2/1 -> magnitude/1
  Gain1/1 -> Product1/1, Product/2
  signal/1 -> Gain1/1
  Sum1/1 -> Mux/1, Fcn/1
  Sum2/1 -> Mux/2, Fcn1/1
  Integ2/1 -> Sum2/1, T2/1
  integ1/1 -> Sum1/1, T1/1
  T2/1 -> Sum2/2
  T1/1 -> Sum1/2
  Product1/1 -> Integ2/1
  Product/1 -> integ1/1
  cos(nwt)/1 -> Product1/2
  sin(nwt)/1 -> Product/1
  Fcn3/1 -> angle/1
  Mux/1 -> Fcn3/1
  Fcn1/1 -> Sum/2
  Fcn/1 -> Sum/1
  Sum/1 -> Fcn2/1

== system systemOffLine/Distance Relay Substation A2/Analog filtering, signal  conditioning/VOLTAGES/Phasor VC ==
  signal : Inport
  Fcn : Fcn  Expr=u^2
  Fcn1 : Fcn  Expr=u^2
  Fcn2 : Fcn  Expr=sqrt(u)
  Fcn3 : Fcn  Expr=180/pi*atan2(u[2],u[1])
  Gain1 : Gain  Gain=k*f1  SaturateOnIntegerOverflow=on  OutDataTypeStr=Inherit: Same as input  ParamDataTypeStr=Inherit: Same as input
  Integ2 : Integrator
  Mux : Mux  Inputs=2
  Product : Product  SaturateOnIntegerOverflow=on  InputSameDT=on  OutDataTypeStr=Inherit: Same as first input
  Product1 : Product  SaturateOnIntegerOverflow=on  InputSameDT=on  OutDataTypeStr=Inherit: Same as first input
  Sum : Sum  SaturateOnIntegerOverflow=on  InputSameDT=on  OutDataTypeStr=Inherit: Same as first input
  Sum1 : Sum  Inputs=+-  SaturateOnIntegerOverflow=on  InputSameDT=on  OutDataTypeStr=Inherit: Same as first input
  Sum2 : Sum  Inputs=+-  SaturateOnIntegerOverflow=on  InputSameDT=on  OutDataTypeStr=Inherit: Same as first input
  T1 : TransportDelay  DelayTime=1/f1  BufferSize=15360
  T2 : TransportDelay  DelayTime=1/f1  BufferSize=15360
  cos(nwt) : Sin  Frequency=2*pi*n*f1  Phase=pi/2  SampleTime=0
  integ1 : Integrator
  sin(nwt) : Sin  Frequency=2*pi*n*f1  SampleTime=0
  magnitude : Outport  InitialOutput=0
  angle : Outport  Port=2  InitialOutput=0
  wires:
  Sum/1 -> Fcn2/1
  Fcn/1 -> Sum/1
  Fcn1/1 -> Sum/2
  Mux/1 -> Fcn3/1
  Fcn3/1 -> angle/1
  sin(nwt)/1 -> Product/1
  cos(nwt)/1 -> Product1/2
  Product/1 -> integ1/1
  Product1/1 -> Integ2/1
  T1/1 -> Sum1/2
  T2/1 -> Sum2/2
  integ1/1 -> T1/1, Sum1/1
  Integ2/1 -> T2/1, Sum2/1
  Sum2/1 -> Fcn1/1, Mux/2
  Sum1/1 -> Fcn/1, Mux/1
  signal/1 -> Gain1/1
  Gain1/1 -> Product/2, Product1/1
  Fcn2/1 -> magnitude/1
